simulink model "NonLinear_Model"  (R2014b)
settings: Solver=ode45  StartTime=0.0  StopTime=600  RelTol=1e-6
settings Model: Creator=NagyZe  LastModifiedBy=NagyZe

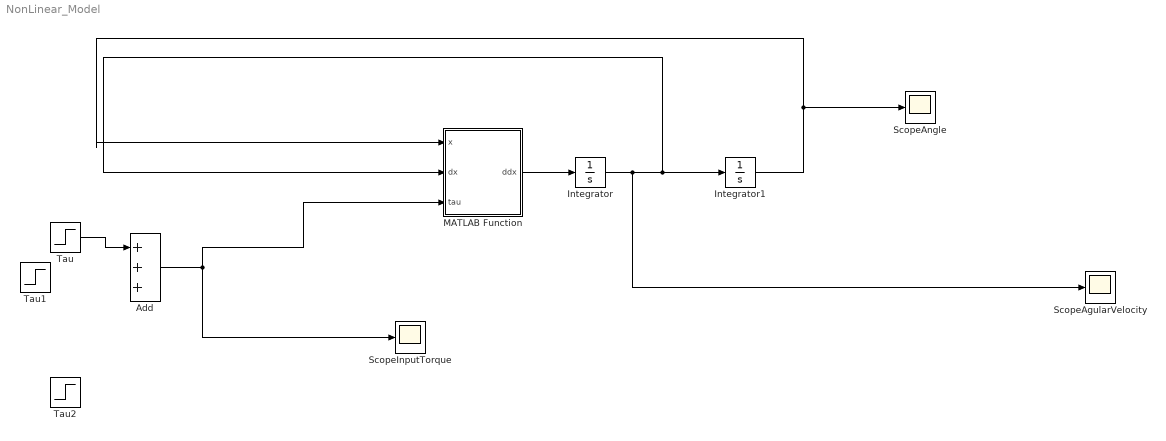
== system NonLinear_Model ==
  Add : Sum  Inputs=+++
  Integrator : Integrator  InitialCondition=[0 0 0]
  Integrator1 : Integrator  InitialCondition=[0 pi 0.1]
  MATLAB Function : MATLAB Function  TreatAsAtomicUnit=on
  ScopeAgularVelocity : Scope
      settings: SaveName=jointVelocity
  ScopeAngle : Scope
      settings: SaveName=jointVelocity1
  ScopeInputTorque : Scope
      settings: SaveName=jointVelocity2
  Tau : Step  Before=[0 1 0]  After=[0 0 0]  SampleTime=0
  Tau1 : Step  Time=80  Before=[0 0 0]  After=[-0.1 0 0]  SampleTime=0
  Tau2 : Step  Time=81  Before=[0 0 0]  After=[0.1 0 0]  SampleTime=0
  wires:
  MATLAB Function/1(ddx) -> Integrator/1
  Integrator/1 -> ScopeAgularVelocity/1, MATLAB Function/2(dx), Integrator1/1
  Integrator1/1 -> ScopeAngle/1, MATLAB Function/1(x)
  Add/1 -> ScopeInputTorque/1, MATLAB Function/3(tau)
  Tau/1 -> Add/1

== matlab function NonLinear_Model/MATLAB Function ==
  data: x input; ddx output; dx input; tau input
function ddx = fcn(x,dx,tau)
%getting the state spacemodel of the system
%give real values to the angles and the angular velocities

%giving some random data for M, L, I
L1=1.25;
L2=1.04;
L3=1.4;
M1=0.91; M2=0.61; M3=0.4;
I1x=1.1; I1y=1.2;I1z=1.3;
I2x=1; I2y=1.1; I2z=1.2;
I3x=1.2; I3y=1; I3z=1.1;
g=9.8;


q1=x(1);
q2=x(2);
q3=x(3);

dq1=dx(1);
dq2=dx(2);
dq3=dx(3);

M=[ I1z + cos(q2)*(sin(q3)*((M3*cos(q2)*sin(q3)*L3^2)/4 + I3y*cos(q2)*sin(q3)) + I2x*cos(q2) + I3x*cos(q2)*cos(q3)^2) + sin(q2)*(I2y*sin(q2) + I3z*sin(q2) + (L2^2*M2*sin(q2))/4 + (L3*M3*((L3*sin(q2))/2 + L2*cos(q3)*sin(q2)))/2 + L2*M3*cos(q3)*((L3*sin(q2))/2 + L2*cos(q3)*sin(q2)) + L2^2*M3*sin(q2)*sin(q3)^2),                                   cos(q2)*(sin(q3)*(I3y*cos(q3) + (L3*M3*(L2 + (L3*cos(q3))/2))/2) - I3x*cos(q3)*sin(q3)), -sin(q2)*((M3*L3^2)/4 + (L2*M3*cos(q3)*L3)/2 + I3z)
                                                                                                                                                                                          cos(q3)*((M3*cos(q2)*sin(q3)*L3^2)/4 + I3y*cos(q2)*sin(q3)) - I3x*cos(q2)*cos(q3)*sin(q3) + (L2*L3*M3*cos(q2)*sin(q3))/2, I2z + cos(q3)*(I3y*cos(q3) + (L3*M3*(L2 + (L3*cos(q3))/2))/2) + (L2^2*M2)/4 + I3x*sin(q3)^2 + L2*M3*(L2 + (L3*cos(q3))/2),                                                   0
                                                                                                                                                                                                                                                   - I3z*sin(q2) - (L3*M3*((L3*sin(q2))/2 + L2*cos(q3)*sin(q2)))/2,                                                                                                                         0,                                   (M3*L3^2)/4 + I3z];
 
C=[ - sin(q2)*((L3*M3*(L2*sin(q2)^2*sin(q3) - (L3*cos(q2)^2*cos(q3)*sin(q3))/2))/2 - L2*M3*sin(q3)*((L3*(cos(q2)^2*sin(q3)^2 + sin(q2)^2))/2 + L2*cos(q3)*sin(q2)^2) + I3x*cos(q2)^2*cos(q3)*sin(q3) - I3y*cos(q2)^2*cos(q3)*sin(q3) + L2*M3*cos(q3)*(L2*sin(q2)^2*sin(q3) - (L3*cos(q2)^2*cos(q3)*sin(q3))/2)) - cos(q2)*(sin(q3)*((L3*M3*(L2*cos(q2)*sin(q2) + (L3*cos(q2)*cos(q3)*sin(q2))/2))/2 - I3x*cos(q2)*cos(q3)*sin(q2) + I3z*cos(q2)*cos(q3)*sin(q2)) + cos(q3)*(I3y*cos(q2)*sin(q2)*sin(q3) - I3z*cos(q2)*sin(q2)*sin(q3))), -sin(q2)*((L3*M3*(L2*sin(q3) + (L3*cos(q3)*sin(q3))/2))/2 - I3x*cos(q3)*sin(q3) + I3y*cos(q3)*sin(q3) + L2*M3*cos(q3)*(L2*sin(q3) + (L3*cos(q3)*sin(q3))/2) - L2*M3*sin(q3)*(L2*cos(q3) + (L3*cos(q3)^2)/2)), (L2*L3*M3*sin(q2)*sin(q3))/2
                                                                                                                                                                                sin(q3)*(I3y*cos(q2)*sin(q2)*sin(q3) - I3z*cos(q2)*sin(q2)*sin(q3)) - cos(q3)*((L3*M3*(L2*cos(q2)*sin(q2) + (L3*cos(q2)*cos(q3)*sin(q2))/2))/2 - I3x*cos(q2)*cos(q3)*sin(q2) + I3z*cos(q2)*cos(q3)*sin(q2)) + I2x*cos(q2)*sin(q2) - I2y*cos(q2)*sin(q2) - L2*M3*(L2*cos(q2)*sin(q2) + (L3*cos(q2)*cos(q3)*sin(q2))/2) - (L2^2*M2*cos(q2)*sin(q2))/4,                                                                                                                                                                                                            0,                            0
                                                                                                                                                                                                                                                                                                                                                                                                (L3*M3*(L2*sin(q2)^2*sin(q3) - (L3*cos(q2)^2*cos(q3)*sin(q3))/2))/2 + I3x*cos(q2)^2*cos(q3)*sin(q3) - I3y*cos(q2)^2*cos(q3)*sin(q3),                                                                                                                  (L3*M3*(L2*sin(q3) + (L3*cos(q3)*sin(q3))/2))/2 - I3x*cos(q3)*sin(q3) + I3y*cos(q3)*sin(q3),                            0];
 

B =[ dq2*(sin(q2)*(I2z*cos(q2) - I2x*cos(q2) + (L3*M3*(L2*cos(q2)*cos(q3) + (L3*cos(q2)*cos(q3)^2)/2 - (L3*cos(q2)*sin(q3)^2)/2))/2 + (L2^2*M2*cos(q2))/4 - I3x*cos(q2)*cos(q3)^2 + I3y*cos(q2)*cos(q3)^2 + I3x*cos(q2)*sin(q3)^2 - I3y*cos(q2)*sin(q3)^2 + L2*M3*sin(q3)*(L2*cos(q2)*sin(q3) + L3*cos(q2)*cos(q3)*sin(q3)) + L2*M3*cos(q3)*(L2*cos(q2)*cos(q3) + (L3*cos(q2)*cos(q3)^2)/2 - (L3*cos(q2)*sin(q3)^2)/2)) - cos(q2)*(cos(q3)*(I3y*cos(q3)*sin(q2) - I3z*cos(q3)*sin(q2)) - I2y*sin(q2) + I2z*sin(q2) - sin(q3)*((M3*sin(q2)*sin(q3)*L3^2)/4 - I3x*sin(q2)*sin(q3) + I3z*sin(q2)*sin(q3)))) - dq3*(cos(q2)*(cos(q3)*(I3x*cos(q3)*sin(q2) - I3y*cos(q2)*sin(q3) + I3z*cos(q2)*sin(q3)) - sin(q3)*((L3*M3*((L3*cos(q2)*cos(q3))/2 - (L3*sin(q2)*sin(q3))/2))/2 - I3x*cos(q2)*cos(q3) + I3z*cos(q2)*cos(q3) - I3y*sin(q2)*sin(q3))) - sin(q2)*(I3z*cos(q2) + (L3^2*M3*cos(q2))/4 - L2*L3*M3*sin(q2)*sin(q3) + (L2*L3*M3*cos(q2)*cos(q3))/2)),                 dq3*cos(q2)*(cos(q3)*(I3y*cos(q3) - I3z*cos(q3)) - sin(q3)*((M3*sin(q3)*L3^2)/4 - I3x*sin(q3) + I3z*sin(q3))), 0
                                                                                                                                                                                                                                                                                                                                                                                                                                                                                dq2*(sin(q3)*(I3y*cos(q3)*sin(q2) - I3z*cos(q3)*sin(q2)) + cos(q3)*((M3*sin(q2)*sin(q3)*L3^2)/4 - I3x*sin(q2)*sin(q3) + I3z*sin(q2)*sin(q3)) + (L2*L3*M3*sin(q2)*sin(q3))/2) + dq3*(sin(q3)*(I3x*cos(q3)*sin(q2) - I3y*cos(q2)*sin(q3) + I3z*cos(q2)*sin(q3)) + cos(q3)*((L3*M3*((L3*cos(q2)*cos(q3))/2 - (L3*sin(q2)*sin(q3))/2))/2 - I3x*cos(q2)*cos(q3) + I3z*cos(q2)*cos(q3) - I3y*sin(q2)*sin(q3)) + L2*M3*((L3*cos(q2)*cos(q3))/2 - (L3*sin(q2)*sin(q3))/2)), -dq3*(sin(q3)*(I3y*cos(q3) - I3z*cos(q3)) + cos(q3)*((M3*sin(q3)*L3^2)/4 - I3x*sin(q3) + I3z*sin(q3)) + (L2*L3*M3*sin(q3))/2), 0
                                                                                                                                                                                                                                                                                                                                                                                                                                                                                                                                                                                                                                                                                                            - dq2*((L3*M3*(L2*cos(q2)*cos(q3) + (L3*cos(q2)*cos(q3)^2)/2 - (L3*cos(q2)*sin(q3)^2)/2))/2 - I3x*cos(q2)*cos(q3)^2 + I3y*cos(q2)*cos(q3)^2 + I3x*cos(q2)*sin(q3)^2 - I3y*cos(q2)*sin(q3)^2) - dq3*((M3*cos(q2)*L3^2)/4 + I3z*cos(q2)),                                                                                                                             0, 0];
G=[ 0, - (L2*M2*g*sin(q2))/2 - L2*M3*g*sin(q2) - (L3*M3*g*cos(q3)*sin(q2))/2, -(L3*M3*g*cos(q2)*sin(q3))/2]';
dx=[dx(1) dx(2) dx(3)]';
%evaluating the matrices

ddx = - inv(M)*C*dx.^2 - M\B*dx + M\tau; 

%ddx = - inv(M)*C*dx.^2 - M\B*dx -M\G + M\tau; 


end
